simulink model "seniales_ruido"  (R2021a)
settings: Solver=VariableStepAuto  StartTime=0.0  StopTime=10.0  RelTol=1e-3
libraries: simulink x2, cstblocks x1
settings Model: Creator=Bremdows  LastModifiedBy=Bremdow

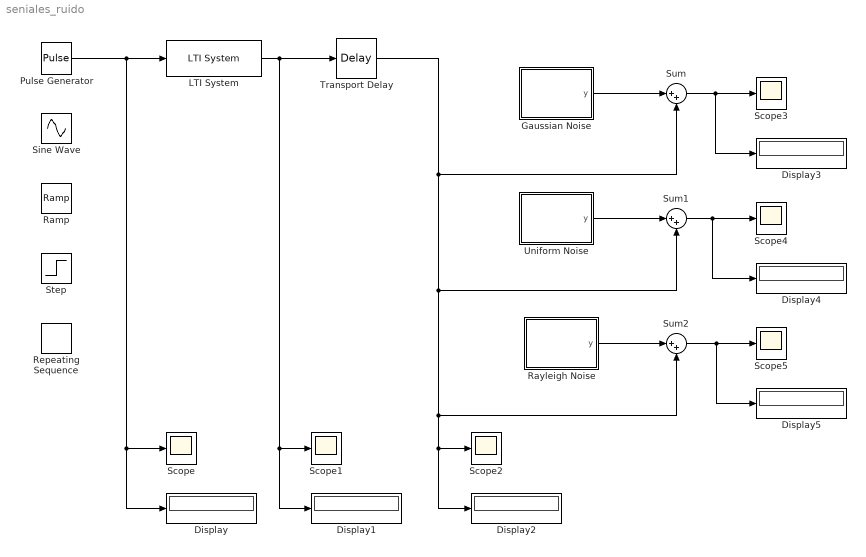
== system seniales_ruido ==
  Display{,1..5} (6 alike) : Display
  Gaussian Noise : MATLAB Function  TreatAsAtomicUnit=on  SystemSampleTime=1  mask{p=1, spf=1, seed=12345}
      mask prompts: p "Power (dBW)"; spf "Samples per frame"
  LTI System : cstblocks/LTI System  sys=tf(1,[1 1])  IC=[]
  Pulse Generator : DiscretePulseGenerator  PulseType=Time based  Period=10  PulseWidth=5
  Ramp : simulink/Sources/Ramp  slope=1  start=0  InitialOutput=0
  Rayleigh Noise : MATLAB Function  TreatAsAtomicUnit=on  SystemSampleTime=1  mask{alpha=1, spf=1, seed=23456}
      mask prompts: alpha "Sigma"; spf "Samples per frame"
  Repeating Sequence : simulink/Sources/Repeating Sequence  rep_seq_t=[0 2]  rep_seq_y=[0 2]
  Scope{,1..5} (6 alike) : Scope
  Sine Wave : Sin  SampleTime=0
  Step : Step  SampleTime=0
  Sum : Sum  Inputs=|++
  Sum1 : Sum  Inputs=|++
  Sum2 : Sum  Inputs=|++
  Transport Delay : TransportDelay
  Uniform Noise : MATLAB Function  TreatAsAtomicUnit=on  SystemSampleTime=1  mask{lb=0, ub=1, spf=1, seed=45678}
      mask prompts: lb "Noise lower bound"; ub "Noise upper bound"; spf "Samples per frame"
  wires:
  Pulse Generator/1 -> Display/1, Scope/1, LTI System/1
  LTI System/1 -> Scope1/1, Display1/1, Transport Delay/1
  Sum/1 -> Display3/1, Scope3/1
  Sum1/1 -> Display4/1, Scope4/1
  Sum2/1 -> Display5/1, Scope5/1
  Transport Delay/1 -> Sum/2, Sum2/2, Display2/1, Scope2/1, Sum1/2
  Uniform Noise/1(y) -> Sum1/1
  Rayleigh Noise/1(y) -> Sum2/1
  Gaussian Noise/1(y) -> Sum/1

== matlab function seniales_ruido/Rayleigh Noise ==
  data: y output; alpha parameter size=[1 1]; spf parameter size=[1 1]; seed parameter size=[1 1]
function y = fcn(alpha,spf, seed)

persistent firstTime

if isempty(firstTime)
  rng(seed);
  firstTime = false;
end

y = abs(alpha*(randn(spf,1)+1i*randn(spf,1)));

== matlab function seniales_ruido/Gaussian Noise ==
  data: y output; p parameter size=[1 1]; spf parameter size=[1 1]; seed parameter size=[1 1]
function y = fcn(p, spf, seed)

persistent firstTime

if isempty(firstTime)
  rng(seed);
  firstTime = false;
end

y = wgn(spf,1,p);

== matlab function seniales_ruido/Uniform Noise ==
  data: y output; ub parameter size=[1 1]; lb parameter size=[1 1]; spf parameter size=[1 1]; seed parameter size=[1 1]
function y = fcn(ub,lb,spf, seed)

persistent firstTime

if isempty(firstTime)
  rng(seed);
  firstTime = false;
end

y = lb + (ub-lb).*rand(spf,1);
